simulink model "plane_control_2019b"  (R2019b)
settings: Solver=FixedStepAuto  StartTime=0.0  StopTime=200  RelTol=1e-3
InitFcn:
  | simin.time = [];
  | simin.signals.values = [10:5:90]';
libraries: mbedblockslib x13, simulink x8
settings Model: SimulationMode=external  SILPILModeSetting=veronly  ExtModeTrigDuration=10  Creator=The MathWorks, Inc.  LastModifiedBy=User
settings SolverCC: PositivePriorityOrder=on
settings DataIOCC: ReturnWorkspaceOutputs=off
settings OptimizationCC: MaxStackSize=64
settings DebuggingCC: ParameterTunabilityLossMsg=error  ArithmeticOperatorsInVariantConditions=warning
settings HardwareCC: ProdBitPerPointer=32  ProdBitPerSizeT=32  ProdBitPerPtrDiffT=32  ProdLargestAtomicInteger=Long  ProdLargestAtomicFloat=Double  ProdWordSize=32  ProdHWDeviceType=ARM Compatible->ARM Cortex  UseEmbeddedCoderFeatures=off
settings ModelReferenceCC: ModelReferenceNumInstancesAllowed=Single
settings SFSimCC: SimUseLocalCustomCode=off  CustomCodeUndefinedFunction=UseInterfaceOnly
settings RTWCC: SystemTargetFile=ert.tlc  HardwareBoard=STM32 Nucleo F767ZI  TemplateMakefile=ert_default_tmf  GenerateReport=on  RTWUseLocalCustomCode=off  Toolchain=GNU Tools for ARM Embedded Processors  LaunchReport=on
settings CodeAppCC: ForceParamTrailComments=on  OperatorAnnotations=on  StateflowObjectComments=on  MATLABSourceComments=on
settings ERTTargetCC: CodeReplacementLibrary=ARM Cortex-M (Optimized)  MultiwordLength=2048  ERTCustomFileBanners=off  SupportContinuousTime=on  SupportNonInlinedSFcns=on  RemoveResetFunc=off  ModelStepFunctionPrototypeControlCompliant=off  ExtMode=on  ExtModeTransport=3  ExtModeStaticAlloc=on  ExtModeStaticAllocSize=2000  ExtModeMexFile=ext_xcp  ExtModeMexArgs=1 3 115200  ExtModeIntrfLevel=Level2 - Open  ERTSrcFileBannerTemplate=codertarget_code_template.cgt  ERTHdrFileBannerTemplate=codertarget_code_template.cgt  ERTDataSrcFileTemplate=codertarget_code_template.cgt  ERTDataHdrFileTemplate=codertarget_code_template.cgt
settings ConfigComp: CovMetricSettings=dsw  CovHtmlReporting=on  CovSaveCumulativeToWorkspaceVar=on  CovSaveSingleToWorkspaceVar=on  CovShowResultsExplorer=off  CovExternalEMLEnable=off

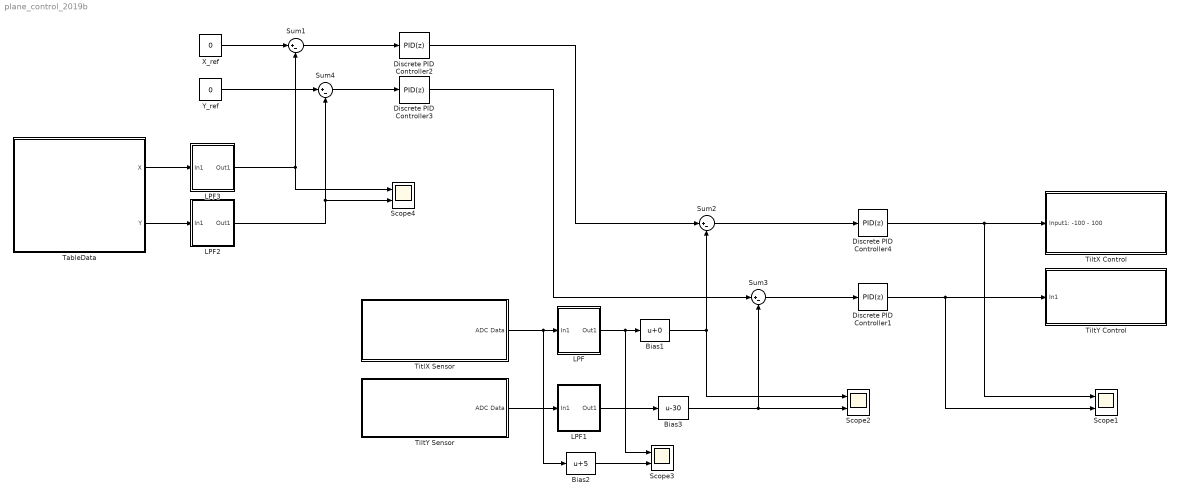
== system plane_control_2019b ==
  Bias1 : Bias
  Bias2 : Bias  Bias=5
  Bias3 : Bias  Bias=-30
  Discrete PID Controller1 : simulink/Continuous/PID Controller  Controller=PID  Form=Parallel  TimeDomain=Discrete-time  SampleTime=5*10^(-3)  IntegratorMethod=Forward Euler  FilterMethod=Forward Euler  ControllerParametersSource=internal  P=2  I=1  D=0.1  UseFilter=off  N=100  TunerSelectOption=Transfer Function Based (PID Tuner App)  InitialConditionSource=internal  InitialConditionForIntegrator=0  InitialConditionForFilter=0  DifferentiatorICPrevScaledInput=0  ExternalReset=none  TrackingMode=off  Kt=1  LimitOutput=off  UpperSaturationLimit=inf  LowerSaturationLimit=-inf  LinearizeAsGain=off  AntiWindupMode=none  Kb=1  POutMin=[]  POutMax=[]  IOutMin=[]  IOutMax=[]  DOutMin=[]  DOutMax=[]  NOutMin=[]  NOutMax=[]  SumOutMin=[]  SumOutMax=[]  SaturationOutMin=[]  SaturationOutMax=[]  PParamMin=[]  PParamMax=[]  IParamMin=[]  IParamMax=[]  DParamMin=[]  DParamMax=[]  NParamMin=[]  NParamMax=[]  KbParamMin=[]  KbParamMax=[]  KtParamMin=[]  KtParamMax=[]  KbOutMin=[]  KbOutMax=[]  KtOutMin=[]  KtOutMax=[]  IntegratorOutMin=[]  IntegratorOutMax=[]  FilterOutMin=[]  FilterOutMax=[]  SumI1OutMin=[]  SumI1OutMax=[]  SumI2OutMin=[]  SumI2OutMax=[]  SumI3OutMin=[]  SumI3OutMax=[]  SumI4OutMin=[]  SumI4OutMax=[]  SumDOutMin=[]  SumDOutMax=[]  DifferentiatorOutMin=[]  DifferentiatorOutMax=[]  FilterDiffOutCoefMin=[]  FilterDiffOutCoefMax=[]  ReciprocalOutMin=[]  ReciprocalOutMax=[]  SumDenOutMin=[]  SumDenOutMax=[]  SumNumOutMin=[]  SumNumOutMax=[]  DivideOutMin=[]  DivideOutMax=[]  IntegratorContinuousStateAttributes=''  IntegratorStateMustResolveToSignalObject=off  IntegratorRTWStateStorageClass=Auto  FilterContinuousStateAttributes=''  FilterStateMustResolveToSignalObject=off  FilterRTWStateStorageClass=Auto  ParallelPVariant=InternalParameters  IdealPVariant=Disabled  IVariant=InternalParameters  DVariant=InternalParameters  IntegratorVariant=Discrete  SatVariant=Disabled  AWVariant=Passthrough  PCopyVariant=Disabled  TRVariant=Disabled  FdbkBlocksVariant=Forward  IdealPFdbkVariant=Disabled  SatFdbkVariant=Disabled  DerivativeFilterVariant=Differentiator  NVariant=Passthrough  NCopyVariant=Disabled_SignalSpec  FilterICVariant=InternalICsDifferentiator  IntegratorICVariant=InternalICs  ExternalResetVariant=Disabled  TRSumVariant=Passthrough  SumFdbkVariant=Disabled  SumVariant=Sum_PID
  Discrete PID Controller2 : simulink/Continuous/PID Controller  Controller=PID  Form=Parallel  TimeDomain=Discrete-time  SampleTime=10*10^(-3)  IntegratorMethod=Forward Euler  FilterMethod=Forward Euler  ControllerParametersSource=internal  P=20  I=1  D=4  UseFilter=off  N=0  TunerSelectOption=Transfer Function Based (PID Tuner App)  InitialConditionSource=internal  InitialConditionForIntegrator=0  InitialConditionForFilter=0  DifferentiatorICPrevScaledInput=0  ExternalReset=none  TrackingMode=off  Kt=1  LimitOutput=off  UpperSaturationLimit=inf  LowerSaturationLimit=-inf  LinearizeAsGain=off  AntiWindupMode=none  Kb=1  POutMin=[]  POutMax=[]  IOutMin=[]  IOutMax=[]  DOutMin=[]  DOutMax=[]  NOutMin=[]  NOutMax=[]  SumOutMin=[]  SumOutMax=[]  SaturationOutMin=[]  SaturationOutMax=[]  PParamMin=[]  PParamMax=[]  IParamMin=[]  IParamMax=[]  DParamMin=[]  DParamMax=[]  NParamMin=[]  NParamMax=[]  KbParamMin=[]  KbParamMax=[]  KtParamMin=[]  KtParamMax=[]  KbOutMin=[]  KbOutMax=[]  KtOutMin=[]  KtOutMax=[]  IntegratorOutMin=[]  IntegratorOutMax=[]  FilterOutMin=[]  FilterOutMax=[]  SumI1OutMin=[]  SumI1OutMax=[]  SumI2OutMin=[]  SumI2OutMax=[]  SumI3OutMin=[]  SumI3OutMax=[]  SumI4OutMin=[]  SumI4OutMax=[]  SumDOutMin=[]  SumDOutMax=[]  DifferentiatorOutMin=[]  DifferentiatorOutMax=[]  FilterDiffOutCoefMin=[]  FilterDiffOutCoefMax=[]  ReciprocalOutMin=[]  ReciprocalOutMax=[]  SumDenOutMin=[]  SumDenOutMax=[]  SumNumOutMin=[]  SumNumOutMax=[]  DivideOutMin=[]  DivideOutMax=[]  IntegratorContinuousStateAttributes=''  IntegratorStateMustResolveToSignalObject=off  IntegratorRTWStateStorageClass=Auto  FilterContinuousStateAttributes=''  FilterStateMustResolveToSignalObject=off  FilterRTWStateStorageClass=Auto  ParallelPVariant=InternalParameters  IdealPVariant=Disabled  IVariant=InternalParameters  DVariant=InternalParameters  IntegratorVariant=Discrete  SatVariant=Disabled  AWVariant=Passthrough  PCopyVariant=Disabled  TRVariant=Disabled  FdbkBlocksVariant=Forward  IdealPFdbkVariant=Disabled  SatFdbkVariant=Disabled  DerivativeFilterVariant=Differentiator  NVariant=Passthrough  NCopyVariant=Disabled_SignalSpec  FilterICVariant=InternalICsDifferentiator  IntegratorICVariant=InternalICs  ExternalResetVariant=Disabled  TRSumVariant=Passthrough  SumFdbkVariant=Disabled  SumVariant=Sum_PID
  Discrete PID Controller3 : simulink/Continuous/PID Controller  Controller=PID  Form=Parallel  TimeDomain=Discrete-time  SampleTime=10*10^(-3)  IntegratorMethod=Forward Euler  FilterMethod=Forward Euler  ControllerParametersSource=internal  P=20  I=1  D=4  UseFilter=off  N=0  TunerSelectOption=Transfer Function Based (PID Tuner App)  InitialConditionSource=internal  InitialConditionForIntegrator=0  InitialConditionForFilter=0  DifferentiatorICPrevScaledInput=0  ExternalReset=none  TrackingMode=off  Kt=1  LimitOutput=off  UpperSaturationLimit=inf  LowerSaturationLimit=-inf  LinearizeAsGain=off  AntiWindupMode=none  Kb=1  POutMin=[]  POutMax=[]  IOutMin=[]  IOutMax=[]  DOutMin=[]  DOutMax=[]  NOutMin=[]  NOutMax=[]  SumOutMin=[]  SumOutMax=[]  SaturationOutMin=[]  SaturationOutMax=[]  PParamMin=[]  PParamMax=[]  IParamMin=[]  IParamMax=[]  DParamMin=[]  DParamMax=[]  NParamMin=[]  NParamMax=[]  KbParamMin=[]  KbParamMax=[]  KtParamMin=[]  KtParamMax=[]  KbOutMin=[]  KbOutMax=[]  KtOutMin=[]  KtOutMax=[]  IntegratorOutMin=[]  IntegratorOutMax=[]  FilterOutMin=[]  FilterOutMax=[]  SumI1OutMin=[]  SumI1OutMax=[]  SumI2OutMin=[]  SumI2OutMax=[]  SumI3OutMin=[]  SumI3OutMax=[]  SumI4OutMin=[]  SumI4OutMax=[]  SumDOutMin=[]  SumDOutMax=[]  DifferentiatorOutMin=[]  DifferentiatorOutMax=[]  FilterDiffOutCoefMin=[]  FilterDiffOutCoefMax=[]  ReciprocalOutMin=[]  ReciprocalOutMax=[]  SumDenOutMin=[]  SumDenOutMax=[]  SumNumOutMin=[]  SumNumOutMax=[]  DivideOutMin=[]  DivideOutMax=[]  IntegratorContinuousStateAttributes=''  IntegratorStateMustResolveToSignalObject=off  IntegratorRTWStateStorageClass=Auto  FilterContinuousStateAttributes=''  FilterStateMustResolveToSignalObject=off  FilterRTWStateStorageClass=Auto  ParallelPVariant=InternalParameters  IdealPVariant=Disabled  IVariant=InternalParameters  DVariant=InternalParameters  IntegratorVariant=Discrete  SatVariant=Disabled  AWVariant=Passthrough  PCopyVariant=Disabled  TRVariant=Disabled  FdbkBlocksVariant=Forward  IdealPFdbkVariant=Disabled  SatFdbkVariant=Disabled  DerivativeFilterVariant=Differentiator  NVariant=Passthrough  NCopyVariant=Disabled_SignalSpec  FilterICVariant=InternalICsDifferentiator  IntegratorICVariant=InternalICs  ExternalResetVariant=Disabled  TRSumVariant=Passthrough  SumFdbkVariant=Disabled  SumVariant=Sum_PID
  Discrete PID Controller4 : simulink/Continuous/PID Controller  Controller=PID  Form=Parallel  TimeDomain=Discrete-time  SampleTime=5*10^(-3)  IntegratorMethod=Forward Euler  FilterMethod=Forward Euler  ControllerParametersSource=internal  P=2  I=1  D=0.1  UseFilter=off  N=100  TunerSelectOption=Transfer Function Based (PID Tuner App)  InitialConditionSource=internal  InitialConditionForIntegrator=0  InitialConditionForFilter=0  DifferentiatorICPrevScaledInput=0  ExternalReset=none  TrackingMode=off  Kt=1  LimitOutput=off  UpperSaturationLimit=inf  LowerSaturationLimit=-inf  LinearizeAsGain=off  AntiWindupMode=none  Kb=1  POutMin=[]  POutMax=[]  IOutMin=[]  IOutMax=[]  DOutMin=[]  DOutMax=[]  NOutMin=[]  NOutMax=[]  SumOutMin=[]  SumOutMax=[]  SaturationOutMin=[]  SaturationOutMax=[]  PParamMin=[]  PParamMax=[]  IParamMin=[]  IParamMax=[]  DParamMin=[]  DParamMax=[]  NParamMin=[]  NParamMax=[]  KbParamMin=[]  KbParamMax=[]  KtParamMin=[]  KtParamMax=[]  KbOutMin=[]  KbOutMax=[]  KtOutMin=[]  KtOutMax=[]  IntegratorOutMin=[]  IntegratorOutMax=[]  FilterOutMin=[]  FilterOutMax=[]  SumI1OutMin=[]  SumI1OutMax=[]  SumI2OutMin=[]  SumI2OutMax=[]  SumI3OutMin=[]  SumI3OutMax=[]  SumI4OutMin=[]  SumI4OutMax=[]  SumDOutMin=[]  SumDOutMax=[]  DifferentiatorOutMin=[]  DifferentiatorOutMax=[]  FilterDiffOutCoefMin=[]  FilterDiffOutCoefMax=[]  ReciprocalOutMin=[]  ReciprocalOutMax=[]  SumDenOutMin=[]  SumDenOutMax=[]  SumNumOutMin=[]  SumNumOutMax=[]  DivideOutMin=[]  DivideOutMax=[]  IntegratorContinuousStateAttributes=''  IntegratorStateMustResolveToSignalObject=off  IntegratorRTWStateStorageClass=Auto  FilterContinuousStateAttributes=''  FilterStateMustResolveToSignalObject=off  FilterRTWStateStorageClass=Auto  ParallelPVariant=InternalParameters  IdealPVariant=Disabled  IVariant=InternalParameters  DVariant=InternalParameters  IntegratorVariant=Discrete  SatVariant=Disabled  AWVariant=Passthrough  PCopyVariant=Disabled  TRVariant=Disabled  FdbkBlocksVariant=Forward  IdealPFdbkVariant=Disabled  SatFdbkVariant=Disabled  DerivativeFilterVariant=Differentiator  NVariant=Passthrough  NCopyVariant=Disabled_SignalSpec  FilterICVariant=InternalICsDifferentiator  IntegratorICVariant=InternalICs  ExternalResetVariant=Disabled  TRSumVariant=Passthrough  SumFdbkVariant=Disabled  SumVariant=Sum_PID
  LPF : Subsystem
  LPF1 : Subsystem
  LPF2 : Subsystem
  LPF3 : Subsystem
  Scope{1..4} (4 alike) : Scope  NumInputPorts=2
  Sum{1..4} (4 alike) : Sum  Inputs=|+-
  TableData : Subsystem
  TiltX Control : Subsystem
  TiltY Control : Subsystem
  "TiltY Sensor " : Subsystem
  TitlX Sensor : Subsystem
  X_ref : Constant  Value=0
  Y_ref : Constant  Value=0
  wires:
  "TiltY Sensor "/1(ADC Data) -> LPF1/1(In1)
  Sum2/1 -> Discrete PID Controller4/1
  Bias1/1 -> Scope2/1, Sum2/2
  TitlX Sensor/1(ADC Data) -> LPF/1(In1), Bias2/1
  Bias3/1 -> Scope2/2, Sum3/2
  Sum3/1 -> Discrete PID Controller1/1
  Discrete PID Controller1/1 -> TiltY Control/1(In1), Scope1/2
  Discrete PID Controller4/1 -> Scope1/1, TiltX Control/1(Input1: -100 - 100)
  LPF/1(Out1) -> Bias1/1, Scope3/1
  Bias2/1 -> Scope3/2
  LPF1/1(Out1) -> Bias3/1
  X_ref/1 -> Sum1/1
  TableData/1(X) -> LPF3/1(In1)
  Y_ref/1 -> Sum4/1
  TableData/2(Y) -> LPF2/1(In1)
  Sum4/1 -> Discrete PID Controller3/1
  Sum1/1 -> Discrete PID Controller2/1
  Discrete PID Controller2/1 -> Sum2/1
  Discrete PID Controller3/1 -> Sum3/1
  LPF2/1(Out1) -> Scope4/2, Sum4/2
  LPF3/1(Out1) -> Sum1/2, Scope4/1

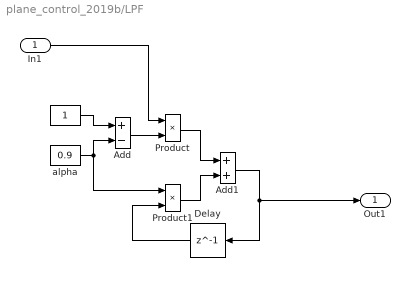
== system plane_control_2019b/LPF ==
  In1 : Inport
  " " : Constant
  Add : Sum  Inputs=+-
  Add1 : Sum
  Delay : Delay  DelayLength=1
  Product : Product
  Product1 : Product
  alpha : Constant  Value=0.9
  Out1 : Outport
  wires:
  Delay/1 -> Product1/2
  Add/1 -> Product/2
  alpha/1 -> Product1/1, Add/2
  Product1/1 -> Add1/2
  Add1/1 -> Out1/1, Delay/1
  In1/1 -> Product/1
  " "/1 -> Add/1
  Product/1 -> Add1/1

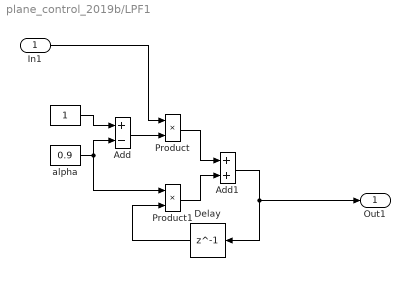
== system plane_control_2019b/LPF1 ==
  In1 : Inport
  " " : Constant
  Add : Sum  Inputs=+-
  Add1 : Sum
  Delay : Delay  DelayLength=1
  Product : Product
  Product1 : Product
  alpha : Constant  Value=0.9
  Out1 : Outport
  wires:
  Product/1 -> Add1/1
  " "/1 -> Add/1
  In1/1 -> Product/1
  Add1/1 -> Delay/1, Out1/1
  Product1/1 -> Add1/2
  alpha/1 -> Add/2, Product1/1
  Add/1 -> Product/2
  Delay/1 -> Product1/2

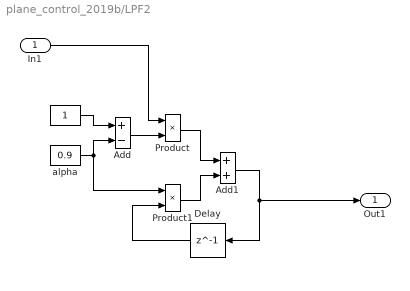
== system plane_control_2019b/LPF2 ==
  In1 : Inport
  " " : Constant
  Add : Sum  Inputs=+-
  Add1 : Sum
  Delay : Delay  DelayLength=1
  Product : Product
  Product1 : Product
  alpha : Constant  Value=0.9
  Out1 : Outport
  wires:
  Delay/1 -> Product1/2
  Add/1 -> Product/2
  alpha/1 -> Product1/1, Add/2
  Product1/1 -> Add1/2
  Add1/1 -> Out1/1, Delay/1
  In1/1 -> Product/1
  " "/1 -> Add/1
  Product/1 -> Add1/1

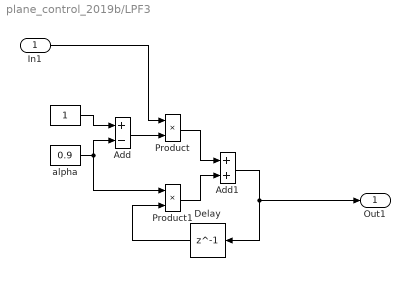
== system plane_control_2019b/LPF3 ==
  In1 : Inport
  " " : Constant
  Add : Sum  Inputs=+-
  Add1 : Sum
  Delay : Delay  DelayLength=1
  Product : Product
  Product1 : Product
  alpha : Constant  Value=0.9
  Out1 : Outport
  wires:
  Product/1 -> Add1/1
  " "/1 -> Add/1
  In1/1 -> Product/1
  Add1/1 -> Delay/1, Out1/1
  Product1/1 -> Add1/2
  alpha/1 -> Add/2, Product1/1
  Add/1 -> Product/2
  Delay/1 -> Product1/2

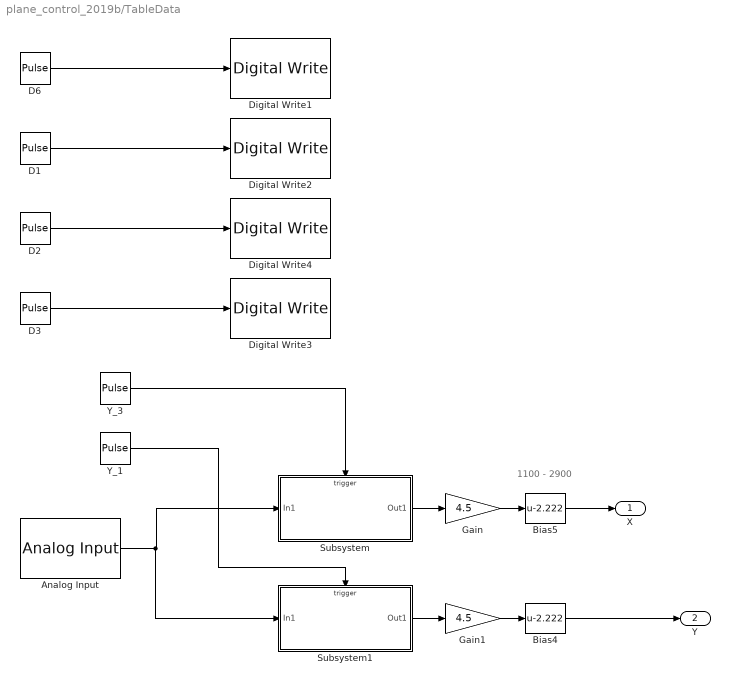
== system plane_control_2019b/TableData ==
  note: 1100 - 2900
  Analog Input : mbedblockslib/Analog Input  Pin=PC_3  ReadResultsOnly=off  ConversionTriggerSource=Software  ExternalTriggerType=uint32( 0 )  OutputDataType=double  EnableConversionCompleteNotify=off  EnableOuputStatus=off  SampleTime=100e-6
      settings: SourceProductName=Simulink Coder Support Package for BBC microbit Board  SourceProductBaseCode=MICROBIT
  Bias4 : Bias  Bias=-2.222
  Bias5 : Bias  Bias=-2.222
  D1 : DiscretePulseGenerator  PulseType=Time based  Period=1000*10^(-6)  PulseWidth=50
  D2 : DiscretePulseGenerator  PulseType=Time based  Period=1000*10^(-6)  PulseWidth=50  PhaseDelay=500*10^(-6)
  D3 : DiscretePulseGenerator  PulseType=Time based  Period=1000*10^(-6)  PulseWidth=50  PhaseDelay=-250*10^(-6)
  D6 : DiscretePulseGenerator  PulseType=Time based  Period=1000*10^(-6)  PulseWidth=50  PhaseDelay=250*10^(-6)
  Digital Write1 : mbedblockslib/Digital Write  Pin=PD_6  Direction=output
      settings: SourceProductName=Simulink Coder Support Package for BBC microbit Board  SourceProductBaseCode=MICROBIT
  Digital Write2 : mbedblockslib/Digital Write  Pin=PD_5  Direction=output
      settings: SourceProductName=Simulink Coder Support Package for BBC microbit Board  SourceProductBaseCode=MICROBIT
  Digital Write3 : mbedblockslib/Digital Write  Pin=PD_3  Direction=output
      settings: SourceProductName=Simulink Coder Support Package for BBC microbit Board  SourceProductBaseCode=MICROBIT
  Digital Write4 : mbedblockslib/Digital Write  Pin=PD_4  Direction=output
      settings: SourceProductName=Simulink Coder Support Package for BBC microbit Board  SourceProductBaseCode=MICROBIT
  Gain : Gain  Gain=4.5
  Gain1 : Gain  Gain=4.5
  Subsystem : Subsystem
  Subsystem1 : Subsystem
  Y_1 : DiscretePulseGenerator  PulseType=Time based  Period=1000*10^(-6)  PhaseDelay=450*10^(-6)
  Y_3 : DiscretePulseGenerator  PulseType=Time based  Period=1000*10^(-6)  PhaseDelay=200*10^(-6)
  X : Outport
  Y : Outport  Port=2
  wires:
  Subsystem1/1(Out1) -> Gain1/1
  Bias4/1 -> Y/1
  D2/1 -> Digital Write4/1
  Analog Input/1 -> Subsystem1/1(In1), Subsystem/1(In1)
  D3/1 -> Digital Write3/1
  Y_1/1 -> Subsystem1/Trigger
  Subsystem/1(Out1) -> Gain/1
  D1/1 -> Digital Write2/1
  D6/1 -> Digital Write1/1
  Gain/1 -> Bias5/1
  Y_3/1 -> Subsystem/Trigger
  Gain1/1 -> Bias4/1
  Bias5/1 -> X/1

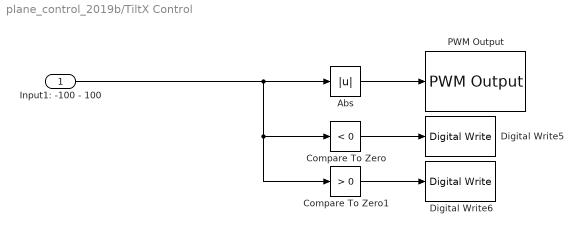
== system plane_control_2019b/TiltX Control ==
  Input1: -100 - 100 : Inport
  Abs : Abs
  Compare To Zero : simulink/Logic and Bit Operations/Compare To Zero  relop=<  OutDataTypeStr=boolean
  Compare To Zero1 : simulink/Logic and Bit Operations/Compare To Zero  relop=>  OutDataTypeStr=boolean
  Digital Write5 : mbedblockslib/Digital Write  Pin=PE_3  Direction=output
      settings: SourceProductName=Simulink Coder Support Package for BBC microbit Board  SourceProductBaseCode=MICROBIT
  Digital Write6 : mbedblockslib/Digital Write  Pin=PF_7  Direction=output
      settings: SourceProductName=Simulink Coder Support Package for BBC microbit Board  SourceProductBaseCode=MICROBIT
  PWM Output : mbedblockslib/PWM Output  Pin=PD_12  EnableInputFrequency=off  InitialFrequency=400  InitialDutyCycle=0  NotificationType=None
      settings: SourceProductName=Simulink Coder Support Package for BBC microbit Board  SourceProductBaseCode=MICROBIT
  wires:
  Compare To Zero/1 -> Digital Write5/1
  Abs/1 -> PWM Output/1
  Input1: -100 - 100/1 -> Abs/1, Compare To Zero1/1, Compare To Zero/1
  Compare To Zero1/1 -> Digital Write6/1

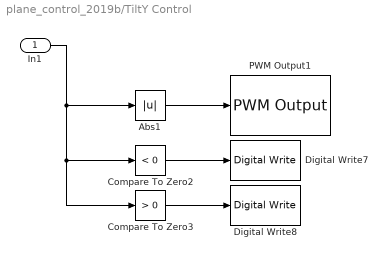
== system plane_control_2019b/TiltY Control ==
  In1 : Inport
  Abs1 : Abs
  Compare To Zero2 : simulink/Logic and Bit Operations/Compare To Zero  relop=<  OutDataTypeStr=boolean
  Compare To Zero3 : simulink/Logic and Bit Operations/Compare To Zero  relop=>  OutDataTypeStr=boolean
  Digital Write7 : mbedblockslib/Digital Write  Pin=PF_8  Direction=output
      settings: SourceProductName=Simulink Coder Support Package for BBC microbit Board  SourceProductBaseCode=MICROBIT
  Digital Write8 : mbedblockslib/Digital Write  Pin=PF_9  Direction=output
      settings: SourceProductName=Simulink Coder Support Package for BBC microbit Board  SourceProductBaseCode=MICROBIT
  PWM Output1 : mbedblockslib/PWM Output  Pin=PD_13  EnableInputFrequency=off  InitialFrequency=400  InitialDutyCycle=0  NotificationType=None
      settings: SourceProductName=Simulink Coder Support Package for BBC microbit Board  SourceProductBaseCode=MICROBIT
  wires:
  Compare To Zero2/1 -> Digital Write7/1
  Compare To Zero3/1 -> Digital Write8/1
  In1/1 -> Compare To Zero3/1, Compare To Zero2/1, Abs1/1
  Abs1/1 -> PWM Output1/1

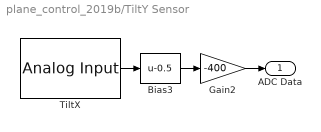
== system plane_control_2019b/TiltY Sensor  ==
  Bias3 : Bias  Bias=-0.5
  Gain2 : Gain  Gain=-400
  TiltX : mbedblockslib/Analog Input  Pin=PF_3  ReadResultsOnly=off  ConversionTriggerSource=Software  ExternalTriggerType=uint32( 0 )  OutputDataType=double  EnableConversionCompleteNotify=off  EnableOuputStatus=off  SampleTime=1*10^(-4)
      settings: SourceProductName=Simulink Coder Support Package for BBC microbit Board  SourceProductBaseCode=MICROBIT
  ADC Data : Outport
  wires:
  Bias3/1 -> Gain2/1
  Gain2/1 -> ADC Data/1
  TiltX/1 -> Bias3/1

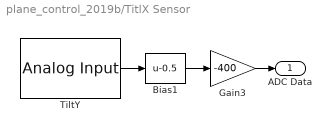
== system plane_control_2019b/TitlX Sensor ==
  Bias1 : Bias  Bias=-0.5
  Gain3 : Gain  Gain=-400
  TiltY : mbedblockslib/Analog Input  Pin=PC_0  ReadResultsOnly=off  ConversionTriggerSource=Software  ExternalTriggerType=uint32( 0 )  OutputDataType=double  EnableConversionCompleteNotify=off  EnableOuputStatus=off  SampleTime=1*10^(-4)
      settings: SourceProductName=Simulink Coder Support Package for BBC microbit Board  SourceProductBaseCode=MICROBIT
  ADC Data : Outport
  wires:
  Gain3/1 -> ADC Data/1
  TiltY/1 -> Bias1/1
  Bias1/1 -> Gain3/1

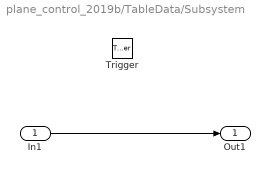
== system plane_control_2019b/TableData/Subsystem ==
  In1 : Inport
  Trigger : TriggerPort  VariantControl=Variant  PortDimensions=1
  Out1 : Outport
  wires:
  In1/1 -> Out1/1

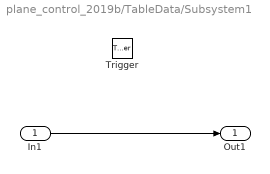
== system plane_control_2019b/TableData/Subsystem1 ==
  In1 : Inport
  Trigger : TriggerPort  VariantControl=Variant  PortDimensions=1
  Out1 : Outport
  wires:
  In1/1 -> Out1/1
